simulink model "fxpdemo_fix2fixinh1"  (Simulink 5.0)
settings: Solver=FixedStepDiscrete  SolverMode=SingleTasking  StartTime=0.0  StopTime=0.9985  FixedStep=0.001  RelTol=1e-3  AbsTol=1e-6
libraries: fixpt_lib_4 x6, fixpt_lib_3p1 x1
settings Model: RequirementInfo=9  CovMetricSettings=d  MinMaxOverflowLogging=MinMaxAndOverflow  Creator=andyb  LastModifiedBy=andyb  ExtModeTrigMode=oneshot  ExtModeArmWhenConnect=off  ExtModeAutoUpdateStatusClock=off  LimitDataPoints=off  IntegerOverflowMsg=none  ParameterDowncastMsg=warning  ParameterOverflowMsg=warning  ParameterPrecisionLossMsg=none  BooleanDataType=off

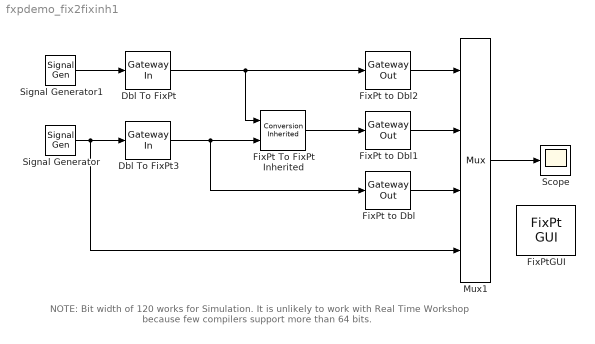
== system fxpdemo_fix2fixinh1 ==
  note: NOTE: Bit width of 120 works for Simulation.  It is unlikely to work with
      | Real Time Workshop because few compilers support more than 64 bits.
  Dbl To FixPt : fixpt_lib_4/Data Type/Gateway In  InRealWorld=Real World Value  OutputDataTypeScalingMode=Specify via dialog  OutDataType=ufix( 4 )  OutScaling=2^(-3)  RndMeth=Nearest  DoSatur=on
  Dbl To FixPt3 : fixpt_lib_4/Data Type/Gateway In  InRealWorld=Real World Value  OutputDataTypeScalingMode=Specify via dialog  OutDataType=sfix(120)  OutScaling=2^(-116)  DoSatur=on
  FixPt To FixPt Inherited : fixpt_lib_4/Data Type/Conversion Inherited  ConvertRealWorld=Real World Value  RndMeth=Nearest  DoSatur=on
  FixPt to Dbl : fixpt_lib_4/Data Type/Gateway Out  OutRealWorld=Real World Value  OutBuiltInType=double  DoSatur=off
  FixPt to Dbl1 : fixpt_lib_4/Data Type/Gateway Out  OutRealWorld=Real World Value  OutBuiltInType=double  DoSatur=off
  FixPt to Dbl2 : fixpt_lib_4/Data Type/Gateway Out  OutRealWorld=Real World Value  OutBuiltInType=double  DoSatur=off
  FixPtGUI : fixpt_lib_3p1/FixPt GUI
  Mux1 : Mux
  Scope : Scope
      settings: TickLabels=on
  Signal Generator : SignalGenerator  WaveForm=sawtooth  Amplitude=5
  Signal Generator1 : SignalGenerator  Frequency=10
  wires:
  Signal Generator1/1 -> Dbl To FixPt/1
  Dbl To FixPt/1 -> FixPt To FixPt Inherited/1, FixPt to Dbl2/1
  Dbl To FixPt3/1 -> FixPt To FixPt Inherited/2, FixPt to Dbl/1
  Signal Generator/1 -> Dbl To FixPt3/1, Mux1/4
  FixPt To FixPt Inherited/1 -> FixPt to Dbl1/1
  FixPt to Dbl1/1 -> Mux1/2
  FixPt to Dbl2/1 -> Mux1/1
  FixPt to Dbl/1 -> Mux1/3
  Mux1/1 -> Scope/1
